simulink model "StateMachine_Incorrect_Nicolas"  (R2022b)
settings: Solver=ode1  StartTime=0.0  StopTime=60  RelTol=1e-3
undefined symbols (not defined in the file or in its folder): sigbuilder_block
settings Model: Creator=jayerdi  LastModifiedBy=pvalle
settings OptimizationCC: ReuseModelBlockBuffer=on

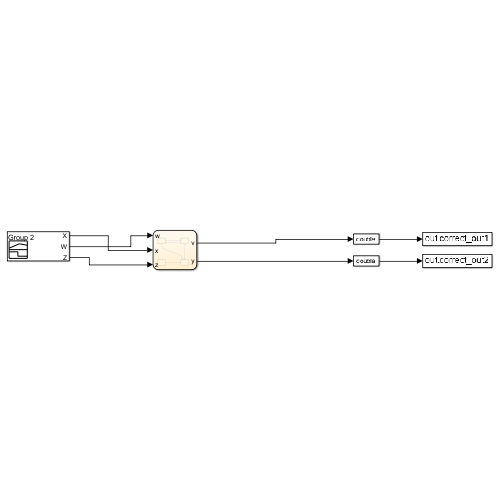
[thumbnail: Simulink's stored preview of the top-level diagram]
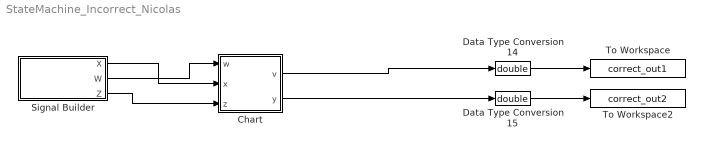
== system StateMachine_Incorrect_Nicolas ==
  Chart : Stateflow chart  TreatAsAtomicUnit=on
  Data Type Conversion14 : DataTypeConversion  OutDataTypeStr=double  SaturateOnIntegerOverflow=off  RndMeth=Floor
  Data Type Conversion15 : DataTypeConversion  OutDataTypeStr=double  SaturateOnIntegerOverflow=off  RndMeth=Floor
  Signal Builder : Subsystem  Tag=STV Subsys  LoadFcn=sigbuilder_block('load');  StartFcn=sigbuilder_block('start');  StopFcn=sigbuilder_block('stop');  ClipboardFcn=sigbuilder_block('clipboard');  mask(Sigbuilder block){tuvar=[0:10]}
      mask help: Simulink:masks:SigbuilderBlock_MD
      mask init:
      | if ~strcmp(get_param(bdroot(gcbh),'SimulationStatus'),'stopped') tuvar = sigbuilder_block('maskInit'); end
      settings: CopyFcn=sigbuilder_block('copy');  DeleteFcn=sigbuilder_block('delete');  ModelCloseFcn=sigbuilder_block('modelClose');  PreSaveFcn=sigbuilder_block('preSave');  PauseFcn=sigbuilder_block('pause');  ContinueFcn=sigbuilder_block('continue');  NameChangeFcn=sigbuilder_block('namechange');  OpenFcn=sigbuilder_block('open',[437.6 199.2 550.4 400 ]);  CloseFcn=sigbuilder_block('close');
      mask Display: plot(0, 0, 100, 100,[2, 2, 32, 32, 2], [68, 8, 8, 68, 68],[32, 2], [38, 38], [32, 19, 2],[53, 60, 44], [32, 17, 17, 2],[16, 16, 31, 31]);txt = getActiveGroup(gcbh);text(2, 100, txt,'verticalAlignment', 'top');
  To Workspace : ToWorkspace  VariableName=correct_out1  SaveFormat=Timeseries  SampleTime=-1
  To Workspace2 : ToWorkspace  VariableName=correct_out2  SaveFormat=Timeseries  SampleTime=-1
  wires:
  Signal Builder/1(X) -> Chart/2(x)
  Signal Builder/2(W) -> Chart/1(w)
  Signal Builder/3(Z) -> Chart/3(z)
  Data Type Conversion15/1 -> To Workspace2/1
  Chart/2(y) -> Data Type Conversion15/1
  Data Type Conversion14/1 -> To Workspace/1
  Chart/1(v) -> Data Type Conversion14/1

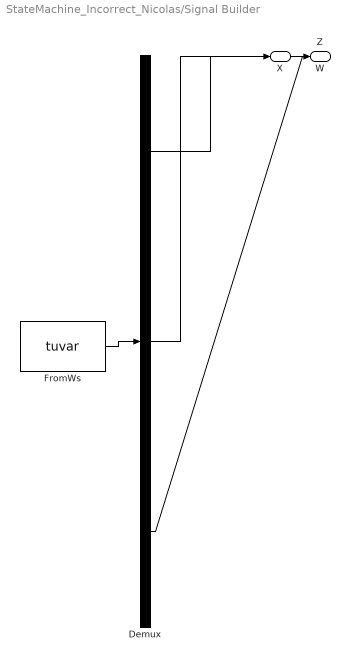
== system StateMachine_Incorrect_Nicolas/Signal Builder ==
  Demux : Demux  Tag=STV Demux  Outputs=3
      settings: DisplayOption=none
  FromWs : FromWorkspace  Tag=STV FromWs  VariableName=tuvar
      SigBuilderData=|
      | common.afterFinalStr = 'Extrapolate'
      | common.sampleTime = 0
      | dataSet(1).timeRange = [0 60]
      | dataSet(1).name = 'Group 1'
      | dataSet(2).timeRange = [0 60]
      | dataSet(2).name = 'Group 2'
      | sbobj.Groups(1).Name = 'Group 1'
      | sbobj.Groups(1).Signals(1).Name = 'X'
      | sbobj.Groups(1).Signals(1).XData = [0 4 4 6 6 60]
      | sbobj.Groups(1).Signals(1).YData = [0 0 1 1 0 0]
      | sbobj.Groups(1).Signals(2).Name = 'W'
      | sbobj.Groups(1).Signals(2).XData = [0 60]
      | sbobj.Groups(1).Signals(2).YData = [4 4]
      | sbobj.Groups(1).Signals(3).Name = 'Z'
      | sbobj.Groups(1).Signals(3).XData = [0 60]
      | sbobj.Groups(1).Signals(3).YData = [10 10]
      | sbobj.Groups(1).TimeRange = [0 60]
      | sbobj.Groups(2).Name = 'Group 2'
      | sbobj.Groups(2).Signals(1).Name = 'X'
      | sbobj.Groups(2).Signals(1).XData = [0 4 4 6 6 60]
      | sbobj.Groups(2).Signals(1).YData = [0 0 1 1 0 0]
      | sbobj.Groups(2).Signals(2).Name = 'W'
      | sbobj.Groups(2).Signals(2).XData = [0 60]
      | sbobj.Groups(2).Signals(2).YData = [2 2]
      | sbobj.Groups(2).Signals(3).Name = 'Z'
      | sbobj.Groups(2).Signals(3).XData = [0 60]
      | sbobj.Groups(2).Signals(3).YData = [10 10]
      | sbobj.Groups(2).TimeRange = [0 60]
  X : Outport  Tag=STV Outport
  W : Outport  Tag=STV Outport  Port=2
  Z : Outport  Tag=STV Outport  Port=3
  wires:
  Demux/1 -> X/1
  FromWs/1 -> Demux/1
  Demux/2 -> W/1
  Demux/3 -> Z/1

== stateflow chart StateMachine_Incorrect_Nicolas/Chart ==
  state State0
    v = 0;
    y = 0;
  state State1
    y = 1;
  state State2
    y = 3;
  state State3
    v = w;
  (default) -> State0
  State0 -> State1 : [w > 3]
  State1 -> State0 [order 2] : [w>5]
  State3 -> State0 : [x == 2]
  State1 -> State3 [order 1] : after(1,sec)
  State2 -> State3 : [z == 0]
  data: w input; x input; z input; v output; y output
